simulink model "BuckBooster_simulink"  (R2020b)
settings: Solver=VariableStepAuto  StartTime=0.0  StopTime=0.04  RelTol=1e-3
undefined symbols (not defined in the file or in its folder): denct, numct
libraries: powerlib x9, cstblocks x1, powerlib_meascontrol x1
settings Model: OrderedModelArguments=off  Creator=leona  LastModifiedBy=LACER-R3

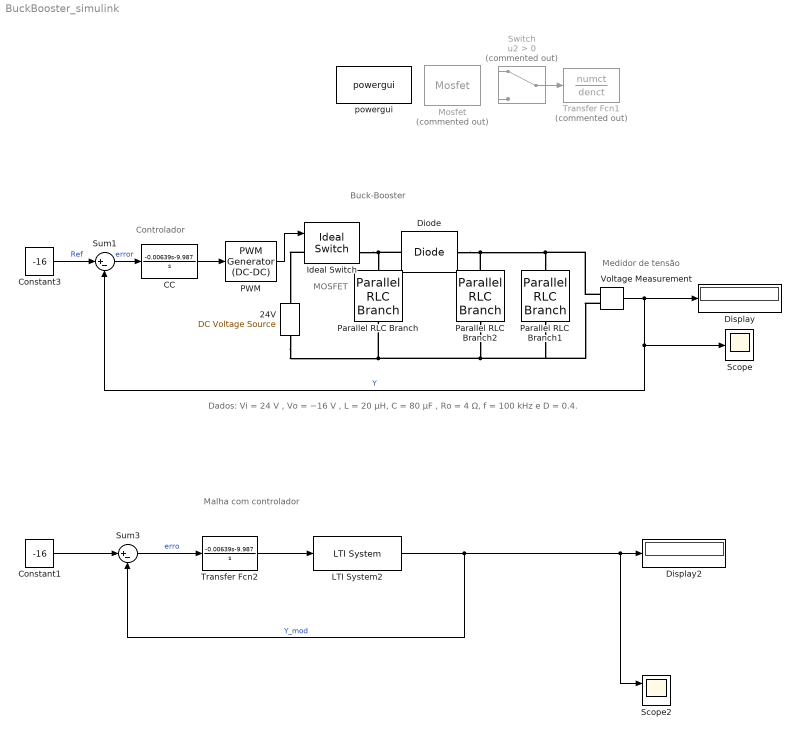
== system BuckBooster_simulink ==
  note: Medidor de tensão
  note: MOSFET
  note: Controlador
  note: Dados: Vi = 24 V , Vo = −16 V , L = 20 μH, C = 80 μF , Ro = 4 Ω, f = 100 kHz e
      | D = 0.4.
  note: Malha com controlador
  note: Buck-Booster
  24V : powerlib/Electrical Sources/DC Voltage Source  Amplitude=24  Measurements=None
  CC : TransferFcn  Numerator=[-0.00639 -9.987]  Denominator=[1 0]
  Constant1 : Constant  Value=-16
  Constant3 : Constant  Value=-16
  Diode : powerlib/Power Electronics/Diode  Ron=0.0  Lon=0  Vf=0.0  IC=0  UseSnubber=0  Rs=0  Cs=0  Measurements=off
  Display : Display
  Display2 : Display
  Ideal Switch : powerlib/Power Electronics/Ideal Switch  Ron=0.001  Lon=0  IC=0  Rs=1e5  Cs=inf  Measurements=on
  LTI System2 : cstblocks/LTI System  sys=Gtfbuckb  IC=[]
  Mosfet : powerlib/Power Electronics/Mosfet  Commented=on  Ron=0.1  Lon=0  Rd=0.01  Vfd=0  IC=0  Rs=1e5  Cs=inf  Measurements=on
  PWM : powerlib_meascontrol/Pulse & Signal Generators/PWM Generator (DC-DC)  Fsw=100000  Ts=0
  Parallel RLC Branch : powerlib/Elements/Parallel RLC Branch  LConnTagsString=a  RConnTagsString=__new0  BranchType=L  Resistance=1  Inductance=20*10^-6  SetiL0=off  InitialCurrent=0  Capacitance=1e-6  Setx0=off  InitialVoltage=0  Measurements=None
  Parallel RLC Branch1 : powerlib/Elements/Parallel RLC Branch  LConnTagsString=a  RConnTagsString=__new0  BranchType=R  Resistance=4  Inductance=1e-3  SetiL0=off  InitialCurrent=0  Capacitance=1e-6  Setx0=off  InitialVoltage=0  Measurements=None
  Parallel RLC Branch2 : powerlib/Elements/Parallel RLC Branch  LConnTagsString=a  RConnTagsString=__new0  BranchType=C  Resistance=4  Inductance=1e-3  SetiL0=off  InitialCurrent=0  Capacitance=80*10^-6  Setx0=off  InitialVoltage=0  Measurements=None
  Scope : Scope
  Scope2 : Scope  NumInputPorts=2
  Sum1 : Sum  Inputs=|+-
  Sum3 : Sum  Inputs=|+-
  Switch : Switch  Commented=on  Criteria=u2 > Threshold
  Transfer Fcn1 : TransferFcn  Commented=on  Numerator=numct  Denominator=denct
  Transfer Fcn2 : TransferFcn  Numerator=[-0.00639 -9.987]  Denominator=[1 0]
  Voltage Measurement : powerlib/Measurements/Voltage Measurement  PhasorSimulation=off  OutputType=Complex  PSBequivalent=0
  powergui : powerlib/powergui  Priority=1  SimulationMode=Continuous  SampleTime=50e-6  frequency=60  Iterations=50  frequencyindice=0  Pbase=100e6  ErrMax=1e-4  UnitsV=kV  UnitsW=MW  buscounter=0  FunctionMessages=off  echomessages=off  EnableUseOfTLC=off  CurrentSourceSwitches=off  DisableSnubberDevices=off  DisableRonSwitches=off  DisableVfSwitches=off  DisplayEquations=off  AutomaticDiscreteSolvers=off  SolverType=Tustin/Backward Euler (TBE)  Interpol=off  ExternalGateDelay=off  methode=off  Ts=100  x0status=blocks  SPID=on  SwTol=0  HookPort=off  NonlinearTolerance=1e-4  nMaxIteration=100  ContinueOnMaxIteration=off  RestoreLinks=warning  ResistiveCurrentMeasurement=off  Frange=[0:2:500]  Ylog=off  Xlog=on  ShowGrid=off  save=off  variable=ZData  structure=0  ZoomFFT=off  StartTime=0.0  cycles=1  DisplayStyle=1  fundamental=60  FreqAxis=off  MaxFrequency=1000  frequencyindicesteady=1  RmsSteady=1  display=off
  wires:
  CC/1 -> PWM/1
  Voltage Measurement/1 -> Sum1/2, Scope/1, Display/1  "Y"
  LTI System2/1 -> Sum3/2, Scope2/1, Display2/1  "Y_mod"
  PWM/1 -> Ideal Switch/1
  Sum1/1 -> CC/1  "error"
  Constant1/1 -> Sum3/1
  Sum3/1 -> Transfer Fcn2/1  "erro"
  Transfer Fcn2/1 -> LTI System2/1
  Switch/1 -> Transfer Fcn1/1
  Constant3/1 -> Sum1/1  "Ref"
  connections:
  Parallel RLC Branch2/LConn1 -- Voltage Measurement/LConn1 -- Parallel RLC Branch1/LConn1 -- Diode/LConn1
  24V/LConn1 -- Parallel RLC Branch1/RConn1 -- Voltage Measurement/LConn2 -- Parallel RLC Branch2/RConn1 -- Parallel RLC Branch/RConn1
  Ideal Switch/LConn1 -- 24V/RConn1
  Diode/RConn1 -- Ideal Switch/RConn1 -- Parallel RLC Branch/LConn1
